simulink model "feedback_y"  (R2018b)
settings: Solver=VariableStepAuto  StartTime=0.0  StopTime=10  RelTol=1e-3
undefined symbols (not defined in the file): Ay, Ay_prime, By, By_prime, Cy, Cy_prime, Dy, Dy_prime, Ky, Sy, x0_chap, x0y
settings Model: Creator=Rafik  LastModifiedBy=Rafik

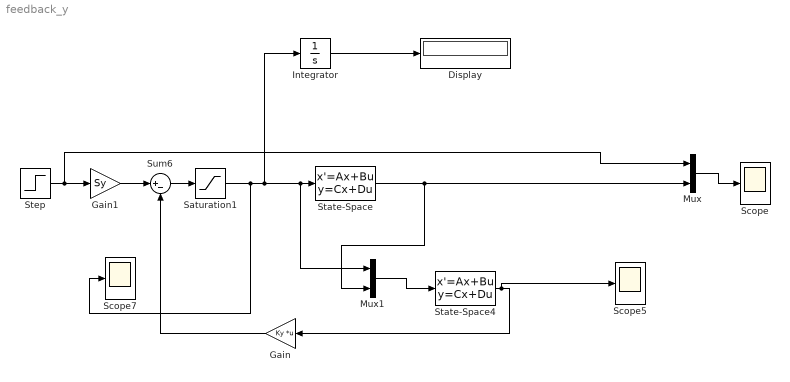
== system feedback_y ==
  Display : Display
  Gain : Gain  Gain=Ky  Multiplication=Matrix(K*u)
  Gain1 : Gain  Gain=Sy
  Integrator : Integrator
  Mux : Mux  Inputs=2
  Mux1 : Mux  Inputs=2
  Saturation1 : Saturate  UpperLimit=110  LowerLimit=-110
  Scope : Scope
  Scope5 : Scope
  Scope7 : Scope
  State-Space : StateSpace  A=Ay  B=By  C=Cy  D=Dy  InitialCondition=x0y
  State-Space4 : StateSpace  A=Ay_prime  B=By_prime  C=Cy_prime  D=Dy_prime  InitialCondition=x0_chap
  Step : Step  Time=0  After=0.5  SampleTime=0
  Sum6 : Sum  Inputs=|+-
  wires:
  Sum6/1 -> Saturation1/1
  Step/1 -> Mux/1, Gain1/1
  Gain/1 -> Sum6/2
  Mux1/1 -> State-Space4/1
  State-Space4/1 -> Scope5/1, Gain/1
  State-Space/1 -> Mux/2, Mux1/2
  Mux/1 -> Scope/1
  Gain1/1 -> Sum6/1
  Saturation1/1 -> Scope7/1, Mux1/1, State-Space/1, Integrator/1
  Integrator/1 -> Display/1
